simulink model "A421_example"  (R2022b)
settings: Solver=VariableStepAuto  StartTime=0.0  StopTime=10.0  RelTol=1e-3
undefined symbols (not defined in the file or in its folder): w_n, z
settings Model: Creator=willb  LastModifiedBy=willb

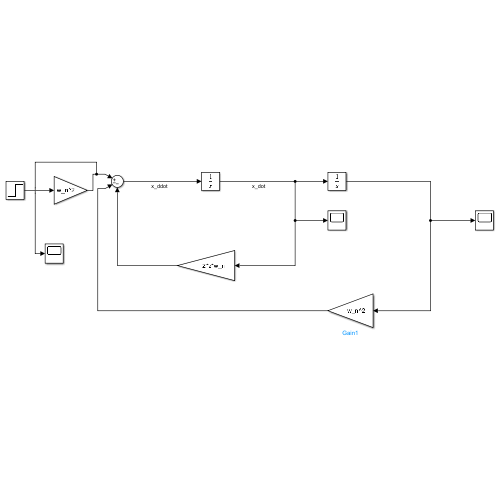
[thumbnail: Simulink's stored preview of the top-level diagram]
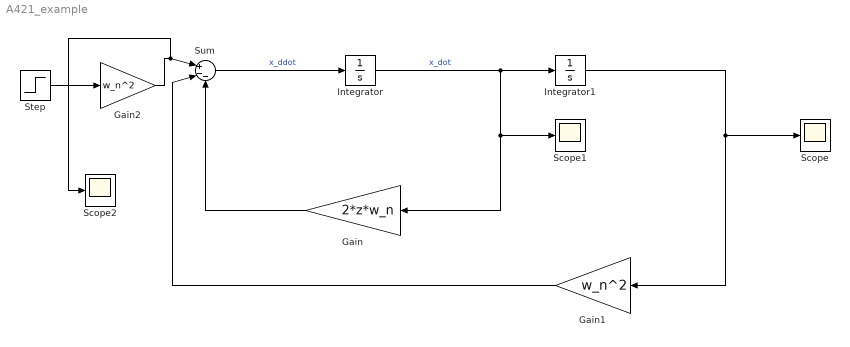
== system A421_example ==
  Gain : Gain  Gain=2*z*w_n
  Gain1 : Gain  Gain=w_n^2
  Gain2 : Gain  Gain=w_n^2
  Integrator : Integrator
  Integrator1 : Integrator
  Scope : Scope
  Scope1 : Scope
  Scope2 : Scope
  Step : Step  SampleTime=0
  Sum : Sum  Inputs=|+--
  wires:
  Sum/1 -> Integrator/1  "x_ddot"
  Integrator/1 -> Gain/1, Scope1/1, Integrator1/1  "x_dot"
  Gain/1 -> Sum/3
  Integrator1/1 -> Scope/1, Gain1/1
  Gain1/1 -> Sum/2
  Gain2/1 -> Scope2/1, Sum/1
  Step/1 -> Gain2/1
